simulink model "ASM_Traffic_V2X_Complete_Model_2"  (R2019a)
settings: Solver=ode1  StartTime=SIM.tstart.v  StopTime=Inf  FixedStep=SIM.StepSize.v  RelTol=1e-3
PostLoadFcn:
  | if any(exist('dsrtsu_mdlpostloadfcn', 'file') ~= 0), dsrtsu_mdlpostloadfcn('Execute', bdroot); end
  | try, asm_mdl_postloadfcn(bdroot, 'UpdateModel', 2200); catch, disp(lasterr); end,
undefined symbols (not defined in the file): _SensorPnts_1, _SensorPnts_13, _SensorPnts_17, _SensorPnts_21, _SensorPnts_25, _SensorPnts_29, _SensorPnts_33, _SensorPnts_37, _SensorPnts_41, _SensorPnts_45, _SensorPnts_49, _SensorPnts_5, _SensorPnts_53, _SensorPnts_57, _SensorPnts_9, _to_, CPT, G5A, ITS, MDL, rad, s_to_rpm, SIM
libraries: simulink x169, ASM_VehicleDynamics_lib x126, ASM_Traffic_lib x83, ASM_Utils_lib x49, mdbs x45, ASM_Environment_lib x17, dspindex x12, dsaV2xLibraryAux x10, dsmpblib x6, dsaV2xAsn1Library x4, dsaV2xLibrary x4, ASM_BrakeHydraulics_lib x4
(part 12 of 36)

== system ASM_Traffic_V2X_Complete_Model_2/MDL/Environment/Maneuver/LastValues ==
  VehicleDynamics_Signals : Inport
  Driver_Signals : Inport  Port=2
  Road_Signals : Inport  Port=3
  Maneuver_RefSignals : Inport  Port=4
  AvoidAlgLoop_AccPed : Memory
  AvoidAlgLoop_BrakePed : Memory
  AvoidAlgLoop_ClutchPed : Memory
  AvoidAlgLoop_Gear : Memory
  AvoidAlgLoop_Steer{,1..4} (5 alike) : Memory
  Bus Creator3 : BusCreator  Inputs=9
  Bus Selector1 : BusSelector  OutputSignals=Steering.Angle_SteeringWheel[deg],Steering.Trq_SteeringWheel[Nm]
  Bus Selector2 : BusSelector  OutputSignals=Pos_AccPedal[%],Pos_BrakePedal[%],Pos_ClutchPedal[%],Gear[],Angle_SteeringWheel[deg],AutomaticTrmCtrlSignals.SelectorLever[-3T|-2P|-1R|0N|1D]
  Bus Selector3 : BusSelector  OutputSignals=Sw_SteeringMode_Maneuver[1Angle|2Trq]
  Bus Selector5 : BusSelector  OutputSignals=Road_ASMVeh.d_Total_Veh_Road[m],Road_ASMVeh.LaneIdx_Total_Veh_Road[]
  Multiport Switch : MultiPortSwitch  Inputs=2
  LastValues : Outport
  wires:
  Bus Selector5/1 -> AvoidAlgLoop_Steer1/1  "<d_Total_Veh_Road[m]>"
  Bus Selector5/2 -> AvoidAlgLoop_Steer2/1  "<LaneIdx_Total_Veh_Road[]>"
  Road_Signals/1 -> Bus Selector5/1
  Driver_Signals/1 -> Bus Selector2/1
  Bus Creator3/1 -> LastValues/1
  AvoidAlgLoop_Steer2/1 -> Bus Creator3/7  "LaneIdx_Total_Veh_Road_Last[]"
  AvoidAlgLoop_Steer1/1 -> Bus Creator3/6  "d_Total_Veh_Road_Last[m]"
  AvoidAlgLoop_Steer/1 -> Bus Creator3/5  "Angle_SteeringWheel_Last[deg]"
  AvoidAlgLoop_Gear/1 -> Bus Creator3/4  "Gear_Last[]"
  AvoidAlgLoop_ClutchPed/1 -> Bus Creator3/3  "Pos_ClutchPedal_Last[%]"
  AvoidAlgLoop_BrakePed/1 -> Bus Creator3/2  "Pos_BrakePedal_Last[%]"
  AvoidAlgLoop_AccPed/1 -> Bus Creator3/1  "Pos_AccPedal_Last[%]"
  Bus Selector2/1 -> AvoidAlgLoop_AccPed/1  "<Pos_AccPedal[%]>"
  Bus Selector2/2 -> AvoidAlgLoop_BrakePed/1  "<Pos_BrakePedal[%]>"
  Bus Selector2/3 -> AvoidAlgLoop_ClutchPed/1  "<Pos_ClutchPedal[%]>"
  Bus Selector2/4 -> AvoidAlgLoop_Gear/1  "<Gear[]>"
  VehicleDynamics_Signals/1 -> Bus Selector1/1
  AvoidAlgLoop_Steer3/1 -> Bus Creator3/8  "Trq_SteeringWheel_Last[Nm]"
  Bus Selector1/2 -> AvoidAlgLoop_Steer3/1  "<Trq_SteeringWheel[Nm]>"
  Bus Selector2/5 -> Multiport Switch/2  "<Angle_SteeringWheel[deg]>"
  Maneuver_RefSignals/1 -> Bus Selector3/1
  Bus Selector3/1 -> Multiport Switch/1  "<Sw_SteeringMode_Maneuver[1Angle|2Trq]>"
  Multiport Switch/1 -> AvoidAlgLoop_Steer/1
  Bus Selector1/1 -> Multiport Switch/3  "<Angle_SteeringWheel[deg]>"
  AvoidAlgLoop_Steer4/1 -> Bus Creator3/9  "SelectorLever_Last[]"
  Bus Selector2/6 -> AvoidAlgLoop_Steer4/1  "<SelectorLever[-3T|-2P|-1R|0N|1D]>"

== system ASM_Traffic_V2X_Complete_Model_2/MDL/Environment/Maneuver/ParkingBrake ==
  Sw_ParkingBrake[0Off|1On] : Inport
  Bus Creator : BusCreator  Inputs=1
  ParkingBrakeSignals : Outport
  wires:
  Sw_ParkingBrake[0Off|1On]/1 -> Bus Creator/1  "Sw_ParkingBrake[0Off|1On]"
  Bus Creator/1 -> ParkingBrakeSignals/1  "ParkingBrakeSignals"

== system ASM_Traffic_V2X_Complete_Model_2/MDL/Environment/Maneuver/ReplaceBrake ==
  RefSignals_In : Inport
  Info : Inport  Port=2
  Bus Creator : BusCreator  Inputs=15
  Bus Selector : BusSelector  OutputSignals=Pos_AccPedal_Maneuver[%],Pos_BrakePedal_Maneuver[%],Pos_ClutchPedal_Maneuver[%],Gear_Maneuver[],Angle_SteeringWheel_Maneuver[deg],v_Vehicle_Ref_Maneuver[m|s],d_Maneuver[m],LaneIdx_Maneuver[],Dist_Def_Maneuver[],v_Vehicle_Ref_Preview_Maneuver[m|s],v_Vehicle_Ref_Preview_State[0Invalid|1CurrentSeg|2NextSeg],Sw_SteeringMode_Maneuver[1Angle|2Trq],Trq_Steering_Maneuver[Nm],SelectorLever_Maneuver[],Dist_Def_Refline_Maneuver[]
  Bus Selector4 : BusSelector  OutputSignals=ManeuverState[]
  Const_Replace_Pos_BrakePedal[%] : Constant  Value=65
  Multiport Switch : MultiPortSwitch  DataPortOrder=Zero-based contiguous  Inputs=2  zeroidx=on
  ReplaceEnable : Subsystem
  RefSignals : Outport
  wires:
  Bus Selector/15 -> Bus Creator/15  "<Dist_Def_Refline_Maneuver[]>"
  Bus Selector/14 -> Bus Creator/14  "<SelectorLever_Maneuver[]>"
  Bus Selector/13 -> Bus Creator/13  "<Trq_Steering_Maneuver[Nm]>"
  Bus Selector/12 -> Bus Creator/12  "<Sw_SteeringMode_Maneuver[1Angle|2Trq]>"
  Bus Selector/11 -> Bus Creator/11  "<v_Vehicle_Ref_Preview_State[0Invalid|1CurrentSeg|2NextSeg]>"
  Bus Selector/10 -> Bus Creator/10  "<v_Vehicle_Ref_Preview_Maneuver[m|s]>"
  Bus Selector/9 -> Bus Creator/9  "<Dist_Def_Maneuver[]>"
  Bus Selector/8 -> Bus Creator/8  "<LaneIdx_Maneuver[]>"
  Bus Selector/7 -> Bus Creator/7  "<d_Maneuver[m]>"
  [TAG_Sw_MasterBrakeCylinder_Mode] -> ReplaceEnable/2(Sw_MasterBrakeCylinder_Mode[1linear|2physical])
  Bus Selector4/1 -> ReplaceEnable/1(ManeuverState)  "<ManeuverState[]>"
  Info/1 -> Bus Selector4/1
  Multiport Switch/1 -> Bus Creator/2  "Pos_BrakePedal_Maneuver[%]"
  Const_Replace_Pos_BrakePedal[%]/1 -> Multiport Switch/3
  Bus Selector/2 -> Multiport Switch/2  "<Pos_BrakePedal_Maneuver[%]>"
  Bus Creator/1 -> RefSignals/1  "RefSignals"
  Bus Selector/6 -> Bus Creator/6  "<v_Vehicle_Ref_Maneuver[m|s]>"
  Bus Selector/5 -> Bus Creator/5  "<Angle_SteeringWheel_Maneuver[deg]>"
  Bus Selector/4 -> Bus Creator/4  "<Gear_Maneuver[]>"
  Bus Selector/3 -> Bus Creator/3  "<Pos_ClutchPedal_Maneuver[%]>"
  Bus Selector/1 -> Bus Creator/1  "<Pos_AccPedal_Maneuver[%]>"
  RefSignals_In/1 -> Bus Selector/1
  ReplaceEnable/1(ReplaceEnable[0Off|1On]) -> Multiport Switch/1

== system ASM_Traffic_V2X_Complete_Model_2/MDL/Environment/Maneuver/ReplaceSelectorLever_Mode ==
  ModeSignals_In : Inport
  Bus Creator : BusCreator  Inputs=10
  Bus Selector : BusSelector  OutputSignals=AccBr_Mode[1Stim|2Driver],GearClutch_Mode[1Stim|2Driver|3OpenClutch|4RefGear],Steer_Mode[1Stim|2Driver|3Fix],Road_Mode[1NoRoad|2Straight|3Circle|4Road],LatDriver[1LatCtrl1|2LatCtrl2],LatCtrl_Mode[1Pos|2Yaw],AdaptVelocityToRoad_Mode[1Off|2On],ForceToRoad_Mode[1Off|2On],CurvatureCalculation_Mode[1Road|2Driver],SelectorLever_Mode[1Stim|2Driver]
  Multiport Switch : MultiPortSwitch  Inputs=2  DiagnosticForDefault=Warning
  Selector1 : Selector  InputPortWidth=4  IndexOptions=Index vector (dialog)  Indices=[3]  OutputSizes=1
  ModeSignals : Outport
  wires:
  Bus Creator/1 -> ModeSignals/1  "ModeSignals"
  ModeSignals_In/1 -> Bus Selector/1
  [TAG_Sw_ManeuverControl] -> Selector1/1
  Bus Selector/1 -> Bus Creator/1  "<AccBr_Mode[1Stim|2Driver]>"
  Bus Selector/2 -> Bus Creator/2  "<GearClutch_Mode[1Stim|2Driver|3OpenClutch|4RefGear]>"
  Bus Selector/3 -> Bus Creator/3  "<Steer_Mode[1Stim|2Driver|3Fix]>"
  Bus Selector/4 -> Bus Creator/4  "<Road_Mode[1NoRoad|2Straight|3Circle|4Road]>"
  Bus Selector/5 -> Bus Creator/5  "<LatDriver[1LatCtrl1|2LatCtrl2]>"
  Bus Selector/6 -> Bus Creator/6  "<LatCtrl_Mode[1Pos|2Yaw]>"
  Bus Selector/7 -> Bus Creator/7  "<AdaptVelocityToRoad_Mode[1Off|2On]>"
  Bus Selector/8 -> Bus Creator/8  "<ForceToRoad_Mode[1Off|2On]>"
  Selector1/1 -> Multiport Switch/1  "Sw_ManualDriving[1ManSched|2Manual]"
  [TAG_SW_SelectorLever_Mode] -> Multiport Switch/3  "SelectorLever_Mode[1Stim|2Driver]"
  Bus Selector/10 -> Multiport Switch/2  "<SelectorLever_Mode[1Stim|2Driver]>"
  Multiport Switch/1 -> Bus Creator/10  "SelectorLever_Mode[1Stim|2Driver]"
  Bus Selector/9 -> Bus Creator/9  "<CurvatureCalculation_Mode[1Road|2Driver]>"

== system ASM_Traffic_V2X_Complete_Model_2/MDL/Environment/Maneuver/Reset _IfModeSwitched ==
  DrvTrnMode : Inport
  TrmMode : Inport  Port=2
  TireMode : Inport  Port=3
  DTC{1..4} (4 alike) : DataTypeConversion  SaturateOnIntegerOverflow=on  RndMeth=Zero
  Gain_DrvTrnMode : Gain  SaturateOnIntegerOverflow=on  OutDataTypeStr=Inherit: Same as input  ParamDataTypeStr=Inherit: Same as input
  Gain_TireMode : Gain  SaturateOnIntegerOverflow=on  OutDataTypeStr=Inherit: Same as input  ParamDataTypeStr=Inherit: Same as input
  Gain_Total : Gain  SaturateOnIntegerOverflow=on  OutDataTypeStr=Inherit: Same as input  ParamDataTypeStr=Inherit: Same as input
  Gain_TrmMode : Gain  SaturateOnIntegerOverflow=on  OutDataTypeStr=Inherit: Same as input  ParamDataTypeStr=Inherit: Same as input
  IgnoreSimulationStart : Subsystem
  LogOp_Reset : Logic  Operator=OR  Inputs=3  AllPortsSameDT=off
  Mem_DrvTrnMode : Memory
  Mem_TireMode : Memory
  Mem_TrmMode : Memory
  RelOp_DrvTrnMode : RelationalOperator  Operator=~=  RndMeth=Nearest
  RelOp_TireMode : RelationalOperator  Operator=~=  RndMeth=Nearest
  RelOp_TrmMode : RelationalOperator  Operator=~=  RndMeth=Nearest
  Sat_DrvTrnMode : Saturate  UpperLimit=3  LowerLimit=1
  Sat_TireMode : Saturate  UpperLimit=2  LowerLimit=1
  Sat_TrmMode : Saturate  UpperLimit=2  LowerLimit=1
  Reset_IfModeSwitched : Outport
  wires:
  DrvTrnMode/1 -> Sat_DrvTrnMode/1
  Sat_DrvTrnMode/1 -> Mem_DrvTrnMode/1, RelOp_DrvTrnMode/2
  Mem_DrvTrnMode/1 -> RelOp_DrvTrnMode/1
  IgnoreSimulationStart/1(Reset_Out) -> Gain_Total/1
  Gain_Total/1 -> Reset_IfModeSwitched/1
  Sat_TrmMode/1 -> RelOp_TrmMode/2, Mem_TrmMode/1
  Mem_TrmMode/1 -> RelOp_TrmMode/1
  Sat_TireMode/1 -> Mem_TireMode/1, RelOp_TireMode/2
  Mem_TireMode/1 -> RelOp_TireMode/1
  TrmMode/1 -> Sat_TrmMode/1
  TireMode/1 -> Sat_TireMode/1
  RelOp_DrvTrnMode/1 -> DTC1/1
  RelOp_TrmMode/1 -> DTC2/1
  RelOp_TireMode/1 -> DTC3/1
  Gain_DrvTrnMode/1 -> LogOp_Reset/1
  Gain_TrmMode/1 -> LogOp_Reset/2
  Gain_TireMode/1 -> LogOp_Reset/3
  LogOp_Reset/1 -> DTC4/1
  DTC1/1 -> Gain_DrvTrnMode/1
  DTC2/1 -> Gain_TrmMode/1
  DTC3/1 -> Gain_TireMode/1
  DTC4/1 -> IgnoreSimulationStart/1(Reset_In)

== system ASM_Traffic_V2X_Complete_Model_2/MDL/Environment/Maneuver/SimulationControl ==
  VehicleDynamics_Signals : Inport
  Bus Selector4 : BusSelector  OutputSignals=VehicleMovement.Positions.Angle_Vehicle_CoorSys_E[x;y;z][deg].Angle_Roll_Vehicle_CoorSys_E[deg],VehicleMovement.Positions.Angle_Vehicle_CoorSys_E[x;y;z][deg].Angle_Pitch_Vehicle_CoorSys_E[deg]
  KeepVehiclePosition : Subsystem
  Keep_VehiclePosition[0|1] : Outport
  wires:
  KeepVehiclePosition/1(Keep_VehiclePosition[0|1]) -> Keep_VehiclePosition[0|1]/1
  Bus Selector4/1 -> KeepVehiclePosition/1(Angle_Roll_Vehicle_CoorSys_E[deg])  "<Angle_Roll_Vehicle_CoorSys_E[deg]>"
  Bus Selector4/2 -> KeepVehiclePosition/2(Angle_Pitch_Vehicle_CoorSys_E[deg])  "<Angle_Pitch_Vehicle_CoorSys_E[deg]>"
  VehicleDynamics_Signals/1 -> Bus Selector4/1

== system ASM_Traffic_V2X_Complete_Model_2/MDL/Environment/Maneuver/StartButton ==
  StartButton_ManSched[0Off|1On] : Inport
  StartButton_Signals_ : Inport  Port=2
  Bus Creator : BusCreator  Inputs=1
  Bus Selector : BusSelector  OutputSignals=Sw_StartButton[0Off|1On],Sw_StartButton_Mode[1Manual|2ManSched]
  Manual : simulink/Logic and Bit Operations/Compare To Constant  relop===  const=1  OutDataTypeStr=boolean
  Switch : Switch  Criteria=u2 ~= 0
  StartButton_Signals : Outport
  wires:
  StartButton_ManSched[0Off|1On]/1 -> Switch/3
  Manual/1 -> Switch/2
  Bus Creator/1 -> StartButton_Signals/1  "StartButtonSignals"
  Switch/1 -> Bus Creator/1  "Sw_StartButton[0Off|1On]"
  Bus Selector/2 -> Manual/1  "<Sw_StartButton_Mode[1Manual|2ManSched]>"
  Bus Selector/1 -> Switch/1  "<Sw_StartButton[0Off|1On]>"
  StartButton_Signals_/1 -> Bus Selector/1

== system ASM_Traffic_V2X_Complete_Model_2/MDL/Environment/Maneuver/Testbench ==
  SW_Testbench[0Off|1On] : Inport
  n_Engine_Set[rpm] : Inport  Port=2
  Bus Creator : BusCreator  Inputs=2
  Testbench : Outport
  wires:
  SW_Testbench[0Off|1On]/1 -> Bus Creator/1  "SW_Testbench[0Off|1On]"
  Bus Creator/1 -> Testbench/1  "Testbench"
  n_Engine_Set[rpm]/1 -> Bus Creator/2  "n_Engine_Set[rpm]"

== system ASM_Traffic_V2X_Complete_Model_2/MDL/Environment/Maneuver/TipShift ==
  SW_TipTronic[-1Down|0Off|1Up] : Inport
  Bus Creator : BusCreator  Inputs=1
  TipShiftSignals : Outport
  wires:
  SW_TipTronic[-1Down|0Off|1Up]/1 -> Bus Creator/1  "SW_TipTronic[-1Down|0Off|1Up]"
  Bus Creator/1 -> TipShiftSignals/1  "TipShiftSignals"

== system ASM_Traffic_V2X_Complete_Model_2/MDL/Environment/Maneuver/VehicleInitStates ==
  note: Set v_x_Init to zero if Keep_VehiclePosition is enabled or the maneuver state is BRAKE or WAIT.
  note: Use v_x_Init from VehicleInitStates_External if the maneuver state is INIT_MANUAL or MANUAL; else use v_x_Init from the maneuver scheduler.
  Keep_VehiclePosition[0|1] : Inport
  ManeuverState[] : Inport  Port=2
  v_Vehicle_Init_Mnv[km|h] : Inport  Port=3
  VehicleInitStates_External : Inport  Port=4
  Bus Creator1 : BusCreator  Inputs=1
  Const_zero_v_x_Init[km|h] : Constant  Value=0  VectorParams1D=off
  Data Type Conversion1 : DataTypeConversion  OutDataTypeStr=double
  Demux : Demux  Outputs=[1 1 1 3]
  Keep_VehiclePosition_enabled : simulink/Logic and Bit Operations/Compare To Constant  relop===  const=1  OutDataTypeStr=uint8  ZeroCross=off
  Logical Operator3 : Logic  Operator=OR  Inputs=3  AllPortsSameDT=off  OutDataTypeStr=boolean
  Logical Operator4 : Logic  Operator=OR  AllPortsSameDT=off  OutDataTypeStr=boolean
  Multiport Switch1 : MultiPortSwitch  DataPortOrder=Zero-based contiguous  Inputs=2  zeroidx=on
  Multiport Switch2 : MultiPortSwitch  DataPortOrder=Zero-based contiguous  Inputs=2  zeroidx=on
  Mux : Mux  Inputs=3
  Mux1 : Mux  Inputs=[3 3]
  State_BRAKE : simulink/Logic and Bit Operations/Compare To Constant  relop===  const=4  OutDataTypeStr=uint8  ZeroCross=off
  State_INIT_MANUAL : simulink/Logic and Bit Operations/Compare To Constant  relop===  const=6  OutDataTypeStr=uint8  ZeroCross=off
  State_MANUAL : simulink/Logic and Bit Operations/Compare To Constant  relop===  const=7  OutDataTypeStr=uint8  ZeroCross=off
  State_WAIT : simulink/Logic and Bit Operations/Compare To Constant  relop===  const=5  OutDataTypeStr=uint8  ZeroCross=off
  Sw_KeepVehiclePosition_Dependency : Gain
  Sw_ManeuverState_Dependency : Gain
  Unit Delay : UnitDelay  SampleTime=-1
  UnitConversion : ASM_Utils_lib/UnitConversion/UnitConversion  Selection=km/h_to_m/s
  VehicleInitStates : Outport
  wires:
  Demux/3 -> Mux/3  "vz"
  Demux/2 -> Mux/2  "vy"
  Bus Creator1/1 -> VehicleInitStates/1  "VehicleInitStates"
  Mux/1 -> UnitConversion/1
  Demux/4 -> Mux1/2  "w_Init[x;y;z][rad|s]"
  ManeuverState[]/1 -> Sw_ManeuverState_Dependency/1
  Unit Delay/1 -> Mux/1  "vx"
  Mux1/1 -> Bus Creator1/1  "q_dt_Vehicle_Init[6x1]"
  Demux/1 -> Multiport Switch2/3
  State_BRAKE/1 -> Logical Operator3/2
  State_WAIT/1 -> Logical Operator3/3
  Sw_ManeuverState_Dependency/1 -> State_BRAKE/1, State_WAIT/1, State_INIT_MANUAL/1, State_MANUAL/1
  Keep_VehiclePosition[0|1]/1 -> Sw_KeepVehiclePosition_Dependency/1
  Sw_KeepVehiclePosition_Dependency/1 -> Keep_VehiclePosition_enabled/1
  Keep_VehiclePosition_enabled/1 -> Logical Operator3/1
  Logical Operator3/1 -> Data Type Conversion1/1
  Data Type Conversion1/1 -> Multiport Switch1/1
  Const_zero_v_x_Init[km|h]/1 -> Multiport Switch1/3
  Multiport Switch2/1 -> Multiport Switch1/2
  Multiport Switch1/1 -> Unit Delay/1
  State_INIT_MANUAL/1 -> Logical Operator4/1
  State_MANUAL/1 -> Logical Operator4/2
  Logical Operator4/1 -> Multiport Switch2/1
  v_Vehicle_Init_Mnv[km|h]/1 -> Multiport Switch2/2
  VehicleInitStates_External/1 -> Demux/1
  UnitConversion/1 -> Mux1/1  "v_Init[x;y;z][m|s]"

== system ASM_Traffic_V2X_Complete_Model_2/MDL/Environment/Road/ASMSignalCollector ==
  SwitchRoad[0BasicRoad|1StandardRoad] : Inport
  Bus Creator : BusCreator  Inputs=11
  Bus Creator1 : BusCreator  Inputs=2
  Bus Selector1 : BusSelector  OutputSignals=Road_Init,Road_ASMVeh,Road_ContactPoints,Road_Preview  OutputAsBus=on
  Bus Selector2 : BusSelector  OutputSignals=Road_Info,Road_TrafficFellows,UserSignals
  Bus Selector4 : BusSelector  OutputSignals=Road_Init,Road_ASMVeh,Road_ContactPoints,Road_Preview
  Switch1 : Switch  Threshold=0.5
  tag scope: ASMBUS_Environment_Road=global
  wires:
  Bus Creator1/1 -> Bus Creator/11  "LaneSensor_Dynamic"
  [ASMBUS_Environment_LaneSensor_Dynamic_Output] -> Bus Creator1/2  "Sensor_Output"
  [ASMBUS_Environment_LaneSensor_Dynamic_Parameters] -> Bus Creator1/1  "Parameters"
  [ASMBUS_Environment_Ambient] -> Bus Creator/10
  [ASMBUS_Environment_Customized_UserSignals] -> Bus Creator/8
  [ASMBUS_Environment_PosVehGPS] -> Bus Creator/9
  Bus Selector2/2 -> Bus Creator/6  "<Road_TrafficFellows>"
  Bus Selector2/3 -> Bus Creator/7  "<UserSignals>"
  Bus Selector2/1 -> Bus Creator/5  "<Road_Info>"
  Bus Selector4/4 -> Bus Creator/4  "<Road_Preview>"
  Bus Selector4/3 -> Bus Creator/3  "<Road_ContactPoints>"
  Bus Selector4/2 -> Bus Creator/2  "<Road_ASMVeh>"
  Bus Selector4/1 -> Bus Creator/1  "<Road_Init>"
  [ASMBUS_Environment_StandardRoad] -> Bus Selector1/1, Bus Selector2/1
  [ASMBUS_Environment_BasicRoads] -> Switch1/3
  Bus Selector1/1 -> Switch1/1
  SwitchRoad[0BasicRoad|1StandardRoad]/1 -> Switch1/2
  Switch1/1 -> Bus Selector4/1
  Bus Creator/1 -> [ASMBUS_Environment_Road]  "Road"

== system ASM_Traffic_V2X_Complete_Model_2/MDL/Environment/Road/Customize_UserSignals ==
  UserSignals_In : Inport
  Bus Creator : BusCreator  Inputs=3
  Bus Selector1 : BusSelector  OutputSignals=User1[],User2[],User3[]
  CustomizedUserSignals : Subsystem
  ASMSignalBus : Outport
  UserSignals_Customized : Outport  Port=2
  wires:
  UserSignals_In/1 -> Bus Selector1/1
  Bus Creator/1 -> UserSignals_Customized/1, ASMSignalBus/1  "UserSignals_Customized"
  Bus Selector1/1 -> CustomizedUserSignals/1(User1[])  "<User1[]>"
  Bus Selector1/2 -> CustomizedUserSignals/2(User2[])  "<User2[]>"
  Bus Selector1/3 -> CustomizedUserSignals/3(User3[])  "<User3[]>"
  CustomizedUserSignals/1(GPS_Method[]) -> Bus Creator/1
  CustomizedUserSignals/2(Const_Offset_Lat[deg]) -> Bus Creator/2
  CustomizedUserSignals/3(Const_Offset_Long[deg]) -> Bus Creator/3

== system ASM_Traffic_V2X_Complete_Model_2/MDL/Environment/Road/SignalRouting ==
  SwitchRoad[0BasicRoad|1StandardRoad] : Inport
  BasicRoad : Inport  Port=2
  StandardRoad : Inport  Port=3
  Info : Inport  Port=4
  TrafficFellows : Inport  Port=5
  UserSignals : Inport  Port=6
  TrafficObject_Data : Inport  Port=7
  Customized_UserSignals : Inport  Port=8
  Pos_Vehicle_GPS[Long;Lat][deg] : Inport  Port=9
  Ambient : Inport  Port=10
  LaneSensor_Dynamic : Inport  Port=11
  Bus Creator3 : BusCreator  Inputs=12
  Bus Selector1 : BusSelector  OutputSignals=Road_Init,Road_ASMVeh,Road_ContactPoints,Road_Preview
  Mapping_CP : Subsystem
  Switch1 : Switch  Threshold=0.5
  Unit Delay : UnitDelay  SampleTime=-1
  Road : Outport
  wires:
  LaneSensor_Dynamic/1 -> Bus Creator3/12
  TrafficObject_Data/1 -> Bus Creator3/8
  TrafficFellows/1 -> Bus Creator3/6
  UserSignals/1 -> Bus Creator3/7
  Pos_Vehicle_GPS[Long;Lat][deg]/1 -> Bus Creator3/10
  Ambient/1 -> Bus Creator3/11
  Customized_UserSignals/1 -> Bus Creator3/9
  BasicRoad/1 -> Switch1/3
  StandardRoad/1 -> Switch1/1
  SwitchRoad[0BasicRoad|1StandardRoad]/1 -> Switch1/2
  Switch1/1 -> Bus Selector1/1
  Bus Creator3/1 -> Road/1  "Road"
  Bus Selector1/2 -> Bus Creator3/2  "<Road_ASMVeh>"
  Bus Selector1/3 -> Mapping_CP/1(In1)  "<Road_ContactPoints>"
  Bus Selector1/4 -> Bus Creator3/4  "<Road_Preview>"
  Info/1 -> Bus Creator3/5
  Mapping_CP/1(Out1) -> Bus Creator3/3  "Road_ContactPoints"
  Bus Selector1/1 -> Unit Delay/1  "<Road_Init>"
  Unit Delay/1 -> Bus Creator3/1  "Road_InitialStates"

== system ASM_Traffic_V2X_Complete_Model_2/MDL/Environment/Road/distance2TargetLaneLines ==
  posVeh_y : Inport
  Input : Inport  Port=2
  Abs{,1..3} (4 alike) : Abs
  Bus Selector : BusSelector  OutputSignals=CurrentLane.LeftSide.Distance_Marker_Left[m],CurrentLane.RightSide.Distance_Marker_Right[m],CurrentLane.Common.LaneID_PrefLane[]
  LeftLine_position : Constant  Value=-5.25
  RightLine_position : Constant  Value=-8.75
  Subtract : Sum  Inputs=+-
  Subtract1 : Sum  Inputs=+-
  LeftLineDistance : Outport
  RightLineDistance : Outport  Port=2
  Right : Outport  Port=3
  Left : Outport  Port=4
  Lane_ID : Outport  Port=5
  wires:
  Input/1 -> Abs1/1, Abs/1
  LeftLine_position/1 -> Abs2/1
  Abs2/1 -> Subtract1/1
  Abs1/1 -> Subtract1/2
  RightLine_position/1 -> Abs3/1
  Abs3/1 -> Subtract/1
  Abs/1 -> Subtract/2
  Subtract/1 -> Right/1
  Subtract1/1 -> Left/1
  posVeh_y/1 -> Bus Selector/1
  Bus Selector/1 -> LeftLineDistance/1  "<Distance_Marker_Left[m]>"
  Bus Selector/2 -> RightLineDistance/1  "<Distance_Marker_Right[m]>"
  Bus Selector/3 -> Lane_ID/1  "<LaneID_PrefLane[]>"

== system ASM_Traffic_V2X_Complete_Model_2/MDL/Environment/Traffic/ASMSignalCollector ==
  Bus Creator1 : BusCreator  Inputs=3
  tag scope: ASMBUS_Environment_Traffic=global
  wires:
  Bus Creator1/1 -> [ASMBUS_Environment_Traffic]  "Traffic"
  [ASMBUS_Environment_Traffic_FellowMovement] -> Bus Creator1/1
  [ASMBUS_Environment_Traffic_ObjectParameters] -> Bus Creator1/2
  [ASMBUS_Environment_Traffic_Sensors] -> Bus Creator1/3

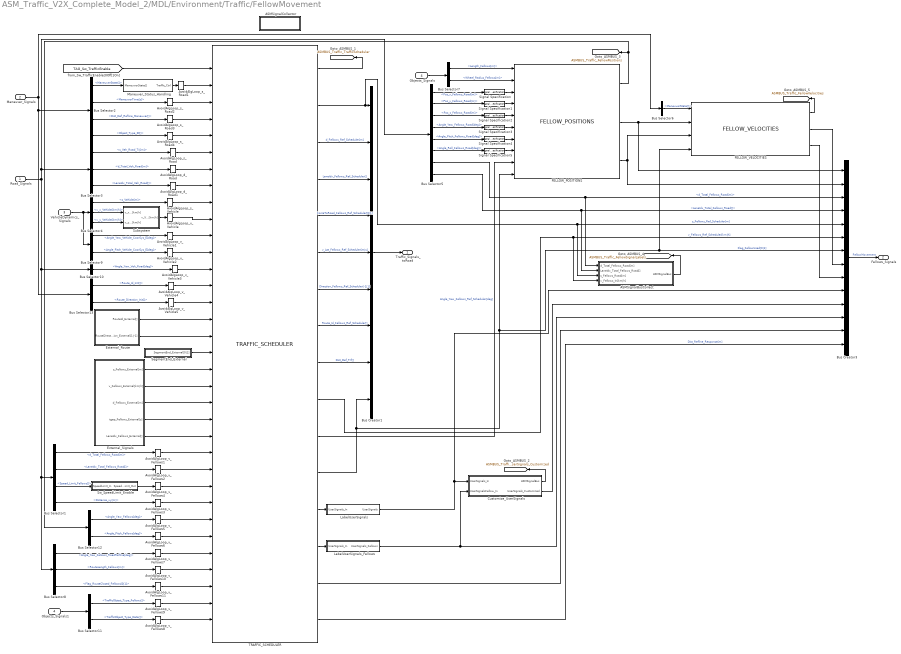
== system ASM_Traffic_V2X_Complete_Model_2/MDL/Environment/Traffic/FellowMovement ==
  Road_Signals : Inport
  Maneuver_Signals : Inport  Port=2
  VehicleDynamics_Signals : Inport  Port=3
  Objects_Signals : Inport  Port=4
  ASMSignalBusCollect : Subsystem
  ASMSignalCollector : Subsystem
  AvoidAlgLoop_d_Road : Memory
  AvoidAlgLoop_d_Road1 : Memory
  AvoidAlgLoop_s_Road{,1..4} (5 alike) : Memory
  AvoidAlgLoop_s_Vehicle : Memory
  AvoidAlgLoop_v_Fellows{1..11} (11 alike) : Memory
  AvoidAlgLoop_v_Vehicle{,1..5} (6 alike) : Memory
  Bus Creator1 : BusCreator  Inputs=9
  Bus Creator3 : BusCreator  Inputs=14
  Bus Selector1 : BusSelector  OutputSignals=Road_TrafficFellows.d_Total_Fellows_Road[m],Road_TrafficFellows.LaneIdx_Total_Fellows_Road[],Road_TrafficFellows.Speed_Limit_Fellows[],Road_TrafficFellows.Dist_Response_Traffic.Distance_xy[m]
  Bus Selector10 : BusSelector  OutputSignals=Road_ASMVeh.Angle_Yaw_Veh_Road[deg]
  Bus Selector11 : BusSelector  OutputSignals=TrafficObject_Type_Fellows[],TrafficObject_Type_Data[]
  Bus Selector12 : BusSelector  OutputSignals=Angle_Fellows[x;y;z][deg].Angle_Yaw_Fellows[deg],Angle_Fellows[x;y;z][deg].Angle_Pitch_Fellows[deg]
  Bus Selector13 : BusSelector  OutputSignals=InitialVehStates.Route_Id_Init[],InitialVehStates.Route_Direction_Init[]
  Bus Selector2 : BusSelector  OutputSignals=Info.ManeuverState[],Info.ManeuverTime[s],RefSignals.Dist_Def_Refline_Maneuver[],Parameters.Object_Type_ID[]
  Bus Selector3 : BusSelector  OutputSignals=Road_ASMVeh.s_Veh_Road_Trj[m],Road_ASMVeh.d_Total_Veh_Road[m],Road_ASMVeh.LaneIdx_Total_Veh_Road[]
  Bus Selector4 : BusSelector  OutputSignals=VehicleMovement.Positions.s_Vehicle[m],VehicleMovement.Velocities.v_x_Vehicle[km|h],VehicleMovement.Velocities.v_y_Vehicle[km|h]
  Bus Selector5 : BusSelector  OutputSignals=Road_TrafficFellows.Pos_x_Fellows_Road[m],Road_TrafficFellows.Pos_y_Fellows_Road[m],Road_TrafficFellows.Pos_z_Fellows_Road[m],Road_TrafficFellows.Angle_Yaw_Fellows_Road[deg],Road_TrafficFellows.Angle_Pitch_Fellows_Road[deg],Road_TrafficFellows.Angle_Roll_Fellows_Road[deg],Road_TrafficFellows.d_Total_Fellows_Road[m],Road_TrafficFellows.LaneIdx_Total_Fellows_Road[]
  Bus Selector6 : BusSelector  OutputSignals=Info.ManeuverState[]
  Bus Selector7 : BusSelector  OutputSignals=FellowsGeometry.Size_Fellows[m].Length_Fellows[m],FellowsGeometry.Wheel_Radius_Fellows[m]
  Bus Selector8 : BusSelector  OutputSignals=Road_TrafficFellows.Angle_Yaw_Fellows_RoadRefline[deg],Road_TrafficFellows.RouteLength_Fellows[m],Road_TrafficFellows.Flag_RouteClosed_Fellows[0|1]
  Bus Selector9 : BusSelector  OutputSignals=VehicleMovement.Positions.Angle_Vehicle_CoorSys_E[x;y;z][deg].Angle_Yaw_Vehicle_CoorSys_E[deg],VehicleMovement.Positions.Angle_Vehicle_CoorSys_E[x;y;z][deg].Angle_Pitch_Vehicle_CoorSys_E[deg]
  Customize_UserSignals : Subsystem
  External_Route : Subsystem
  External_Signals : Subsystem
  FELLOW_POSITIONS : ASM_Traffic_lib/Movement/FELLOW_POSITIONS  StepSize=SIM.StepSize  ASMProperties=struct('Name','FELLOW_POSITIONS','Version','6.0','Library','ASM_Traffic_lib')
  FELLOW_VELOCITIES : ASM_Traffic_lib/Movement/FELLOW_VELOCITIES  ASMProperties=struct('Name','FELLOW_VELOCITIES','Version','1.0','Library','ASM_Traffic_lib')  ASMInstanceName=fellow_velocities  ASMInstanceID=1
  LabelUserSignals : Subsystem
  LabelUserSignals_Fellows : Subsystem
  Maneuver_Status_Handling : Subsystem
  Objects_Signals1 : InportShadow  Port=4
  SegmentEnd_External : Subsystem
  Signal Specification{,1..5} (6 alike) : SignalSpecification  Dimensions=MDL.Traffic.MaxNumFellows.v
  Subsystem : Subsystem
  Sw_SpeedLimit_Enable : Subsystem
  TRAFFIC_SCHEDULER : ASM_Traffic_lib/Movement/TRAFFIC_SCHEDULER  Tag=ASM_SUBCOMPONENT  TrafficVector=MDL.Traffic.TrafficScheduler.Scenario  MaxNumFellows=MDL.Traffic.MaxNumFellows  MaxNumFDUserSignals=MDL.Traffic.MaxNumFDUserSignals  MaxNumUserSignals=MDL.Traffic.MaxNumUserSignals  ASMProperties=struct('Name','TRAFFIC_SCHEDULER','Version','18.0','Library','ASM_Traffic_lib')  ASMInstanceName=traffic_scheduler  ASMInstanceID=1
  Traffic_Signals_toRoad : Outport
  Fellows_Signals : Outport  Port=2
  tag scope: ASMBUS_Traffic_FellowPositions=global, ASMBUS_Traffic_FellowSignalLabels=global, ASMBUS_Traffic_FellowVelocities=global, ASMBUS_Traffic_TrafficScheduler=global, ASMBUS_Traffic_UserSignals_Customized=global
  wires:
  AvoidAlgLoop_v_Fellows9/1 -> TRAFFIC_SCHEDULER/33
  AvoidAlgLoop_v_Fellows11/1 -> TRAFFIC_SCHEDULER/32
  AvoidAlgLoop_v_Fellows10/1 -> TRAFFIC_SCHEDULER/31
  AvoidAlgLoop_v_Fellows7/1 -> TRAFFIC_SCHEDULER/30
  AvoidAlgLoop_v_Fellows6/1 -> TRAFFIC_SCHEDULER/29
  AvoidAlgLoop_v_Fellows5/1 -> TRAFFIC_SCHEDULER/28
  AvoidAlgLoop_v_Fellows3/1 -> TRAFFIC_SCHEDULER/27
  AvoidAlgLoop_v_Fellows4/1 -> TRAFFIC_SCHEDULER/26
  AvoidAlgLoop_v_Fellows2/1 -> TRAFFIC_SCHEDULER/25
  AvoidAlgLoop_v_Fellows1/1 -> TRAFFIC_SCHEDULER/24
  External_Signals/5(LaneIdx_Fellows_External[]) -> TRAFFIC_SCHEDULER/23
  External_Signals/4(tgap_Fellows_External[s]) -> TRAFFIC_SCHEDULER/22
  External_Signals/3(d_Fellows_External[m]) -> TRAFFIC_SCHEDULER/21
  External_Signals/2(v_Fellows_External[km|h]) -> TRAFFIC_SCHEDULER/20
  External_Signals/1(s_Fellows_External[m]) -> TRAFFIC_SCHEDULER/19
  SegmentEnd_External/1(SegmentEnd_External[0|1]) -> TRAFFIC_SCHEDULER/18
  External_Route/2(RouteDirection_External[1|-1]) -> TRAFFIC_SCHEDULER/17
  External_Route/1(RouteId_External[]) -> TRAFFIC_SCHEDULER/16
  Bus Selector13/2 -> AvoidAlgLoop_v_Vehicle5/1  "<Route_Direction_Init[]>"
  AvoidAlgLoop_v_Vehicle5/1 -> TRAFFIC_SCHEDULER/15
  AvoidAlgLoop_s_Road2/1 -> TRAFFIC_SCHEDULER/3
  AvoidAlgLoop_v_Fellows8/1 -> TRAFFIC_SCHEDULER/34
  AvoidAlgLoop_v_Vehicle4/1 -> TRAFFIC_SCHEDULER/14
  Bus Selector8/3 -> AvoidAlgLoop_v_Fellows11/1  "<Flag_RouteClosed_Fellows[0|1]>"
  Bus Selector8/2 -> AvoidAlgLoop_v_Fellows10/1  "<RouteLength_Fellows[m]>"
  AvoidAlgLoop_s_Road4/1 -> TRAFFIC_SCHEDULER/5
  AvoidAlgLoop_s_Road3/1 -> TRAFFIC_SCHEDULER/4
  AvoidAlgLoop_s_Road1/1 -> TRAFFIC_SCHEDULER/2
  AvoidAlgLoop_v_Vehicle3/1 -> TRAFFIC_SCHEDULER/13
  Bus Selector12/2 -> AvoidAlgLoop_v_Fellows6/1  "<Angle_Pitch_Fellows[deg]>"
  FELLOW_POSITIONS/1 -> Bus Selector12/1, [ASMBUS_Traffic_FellowPositions]
  Bus Selector13/1 -> AvoidAlgLoop_v_Vehicle4/1  "<Route_Id_Init[]>"
  Bus Selector10/1 -> AvoidAlgLoop_v_Vehicle3/1  "<Angle_Yaw_Veh_Road[deg]>"
  AvoidAlgLoop_v_Vehicle2/1 -> TRAFFIC_SCHEDULER/12
  AvoidAlgLoop_v_Vehicle1/1 -> TRAFFIC_SCHEDULER/11
  AvoidAlgLoop_v_Vehicle/1 -> TRAFFIC_SCHEDULER/10
  AvoidAlgLoop_s_Vehicle/1 -> TRAFFIC_SCHEDULER/9
  AvoidAlgLoop_d_Road1/1 -> TRAFFIC_SCHEDULER/8
  AvoidAlgLoop_d_Road/1 -> TRAFFIC_SCHEDULER/7
  AvoidAlgLoop_s_Road/1 -> TRAFFIC_SCHEDULER/6
  Bus Selector2/4 -> AvoidAlgLoop_s_Road4/1  "<Object_Type_ID[]>"
  Bus Selector2/3 -> AvoidAlgLoop_s_Road3/1  "<Dist_Def_Refline_Maneuver[]>"
  Bus Selector11/2 -> AvoidAlgLoop_v_Fellows8/1  "<TrafficObject_Type_Data[]>"
  Bus Selector11/1 -> AvoidAlgLoop_v_Fellows9/1  "<TrafficObject_Type_Fellows[]>"
  Objects_Signals1/1 -> Bus Selector11/1
  Bus Selector9/2 -> AvoidAlgLoop_v_Vehicle2/1  "<Angle_Pitch_Vehicle_CoorSys_E[deg]>"
  Bus Selector9/1 -> AvoidAlgLoop_v_Vehicle1/1  "<Angle_Yaw_Vehicle_CoorSys_E[deg]>"
  VehicleDynamics_Signals/1 -> Bus Selector4/1, Bus Selector9/1
  Bus Selector12/1 -> AvoidAlgLoop_v_Fellows5/1  "<Angle_Yaw_Fellows[deg]>"
  Bus Selector8/1 -> AvoidAlgLoop_v_Fellows7/1  "<Angle_Yaw_Fellows_RoadRefline[deg]>"
  TRAFFIC_SCHEDULER/16 -> Bus Creator3/14  "Dist_Refline_Response[m]"
  FELLOW_VELOCITIES/3 -> Bus Creator3/9
  FELLOW_VELOCITIES/2 -> Bus Creator3/8
  Bus Selector6/1 -> FELLOW_VELOCITIES/1  "<ManeuverState[]>"
  FELLOW_VELOCITIES/1 -> [ASMBUS_Traffic_FellowVelocities]
  Subsystem/1(v_Vehicle[km|h]) -> AvoidAlgLoop_v_Vehicle/1
  Bus Selector4/3 -> Subsystem/2(v_y_Vehicle[km|h])  "<v_y_Vehicle[km|h]>"
  Bus Selector4/2 -> Subsystem/1(v_x_Vehicle[km|h])  "<v_x_Vehicle[km|h]>"
  ASMSignalBusCollect/1(ASMSignalBus) -> [ASMBUS_Traffic_FellowSignalLabels]
  TRAFFIC_SCHEDULER/1 -> [ASMBUS_Traffic_TrafficScheduler]
  LabelUserSignals_Fellows/1(UserSignals_Fellows) -> Customize_UserSignals/2(UserSignalsFellow_In), Bus Creator3/12
  LabelUserSignals/1(UserSignals) -> Customize_UserSignals/1(UserSignals_In), Bus Creator3/10
  Customize_UserSignals/2(UserSignals_Customized) -> Bus Creator3/11
  FELLOW_POSITIONS/3 -> Bus Creator3/2, FELLOW_VELOCITIES/3
  FELLOW_POSITIONS/2 -> Bus Creator3/1, FELLOW_VELOCITIES/2
  Bus Selector5/8 -> Bus Creator3/4, ASMSignalBusCollect/2(LaneIdx_Total_Fellows_Road[])  "<LaneIdx_Total_Fellows_Road[]>"
  Bus Selector5/7 -> Bus Creator3/3, ASMSignalBusCollect/1(d_Total_Fellows_Road[m])  "<d_Total_Fellows_Road[m]>"
  TRAFFIC_SCHEDULER/10 -> Bus Creator3/6, ASMSignalBusCollect/4(v_Fellows_In[km|h])  "v_Fellows_Ref_Scheduler[km|h]"
  Customize_UserSignals/1(ASMSignalBus) -> [ASMBUS_Traffic_UserSignals_Customized]
  Objects_Signals/1 -> Bus Selector7/1
  Bus Creator3/1 -> Fellows_Signals/1  "FellowMovement"
  Bus Creator1/1 -> Traffic_Signals_toRoad/1
  Bus Selector7/2 -> FELLOW_POSITIONS/2  "<Wheel_Radius_Fellows[m]>"
  Bus Selector7/1 -> FELLOW_POSITIONS/1  "<Length_Fellows[m]>"
  Bus Selector5/6 -> Signal Specification5/1  "<Angle_Roll_Fellows_Road[deg]>"
  Bus Selector5/5 -> Signal Specification4/1  "<Angle_Pitch_Fellows_Road[deg]>"
  Bus Selector5/4 -> Signal Specification3/1  "<Angle_Yaw_Fellows_Road[deg]>"
  Bus Selector5/3 -> Signal Specification2/1  "<Pos_z_Fellows_Road[m]>"
  Bus Selector5/2 -> Signal Specification1/1  "<Pos_y_Fellows_Road[m]>"
  Bus Selector5/1 -> Signal Specification/1  "<Pos_x_Fellows_Road[m]>"
  TRAFFIC_SCHEDULER/6 -> Bus Creator1/5  "v_Lat_Fellows_Ref_Scheduler[m|s]"
  TRAFFIC_SCHEDULER/5 -> Bus Creator1/4  "ForceToRoad_Fellows_Ref_Scheduler[0|1]"
  TRAFFIC_SCHEDULER/4 -> Bus Creator1/3  "LaneIdx_Fellows_Ref_Scheduler[]"
  TRAFFIC_SCHEDULER/13 -> LabelUserSignals/1(UserSignals_In)
  Bus Selector1/2 -> AvoidAlgLoop_v_Fellows2/1  "<LaneIdx_Total_Fellows_Road[]>"
  Bus Selector1/1 -> AvoidAlgLoop_v_Fellows1/1  "<d_Total_Fellows_Road[m]>"
  Bus Selector3/3 -> AvoidAlgLoop_d_Road1/1  "<LaneIdx_Total_Veh_Road[]>"
  [TAG_Sw_TrafficEnable] -> TRAFFIC_SCHEDULER/1
  Bus Selector4/1 -> AvoidAlgLoop_s_Vehicle/1  "<s_Vehicle[m]>"
  TRAFFIC_SCHEDULER/3 -> Bus Creator1/2  "d_Fellows_Ref_Scheduler[m]"
  TRAFFIC_SCHEDULER/2 -> Bus Creator1/1, Bus Creator3/5, ASMSignalBusCollect/3(s_Fellows_Road[m])  "s_Fellows_Ref_Scheduler[m]"
  Bus Selector3/1 -> AvoidAlgLoop_s_Road/1  "<s_Veh_Road_Trj[m]>"
  Bus Selector2/2 -> AvoidAlgLoop_s_Road2/1  "<ManeuverTime[s]>"
  Bus Selector2/1 -> Maneuver_Status_Handling/1(ManeuverState[])  "<ManeuverState[]>"
  Maneuver_Status_Handling/1(Traffic_Ctrl) -> AvoidAlgLoop_s_Road1/1
  Bus Selector3/2 -> AvoidAlgLoop_d_Road/1  "<d_Total_Veh_Road[m]>"
  Maneuver_Signals/1 -> Bus Selector2/1, Bus Selector13/1, Bus Selector6/1
  Road_Signals/1 -> Bus Selector10/1, Bus Selector1/1, Bus Selector8/1, Bus Selector3/1, Bus Selector5/1
  TRAFFIC_SCHEDULER/7 -> Bus Creator1/6  "Direction_Fellows_Ref_Scheduler[-1|1]"
  TRAFFIC_SCHEDULER/12 -> Bus Creator3/7, FELLOW_VELOCITIES/4, FELLOW_POSITIONS/10, Bus Creator1/9  "Flag_FellowUsed[0|1]"
  TRAFFIC_SCHEDULER/8 -> Bus Creator1/7  "Route_Id_Fellows_Ref_Scheduler[]"
  TRAFFIC_SCHEDULER/9 -> Bus Creator1/8  "Dist_Def_Trf[]"
  Bus Selector1/4 -> AvoidAlgLoop_v_Fellows3/1  "<Distance_xy[m]>"
  Bus Selector1/3 -> Sw_SpeedLimit_Enable/1(SpeedLimit_In)  "<Speed_Limit_Fellows[]>"
  Sw_SpeedLimit_Enable/1(SpeedLimit_Out) -> AvoidAlgLoop_v_Fellows4/1
  Signal Specification/1 -> FELLOW_POSITIONS/3
  Signal Specification1/1 -> FELLOW_POSITIONS/4
  Signal Specification2/1 -> FELLOW_POSITIONS/5
  Signal Specification3/1 -> FELLOW_POSITIONS/6
  Signal Specification4/1 -> FELLOW_POSITIONS/7
  Signal Specification5/1 -> FELLOW_POSITIONS/8
  TRAFFIC_SCHEDULER/14 -> LabelUserSignals_Fellows/1(UserSignals_In)
  TRAFFIC_SCHEDULER/15 -> Bus Creator3/13
  TRAFFIC_SCHEDULER/11 -> FELLOW_POSITIONS/9  "Angle_Yaw_Fellows_Ref_Scheduler[deg]"

== system ASM_Traffic_V2X_Complete_Model_2/MDL/Environment/Traffic/ObjectParameters ==
  Maneuver_Signals : Inport
  ASMSignalCollector : Subsystem
  Bus Creator : BusCreator  Inputs=4
  Bus Creator1 : BusCreator  Inputs=7
  Bus Selector : BusSelector  OutputSignals=MdlControl.RoadControl[]
  DISCRETE_OBJECTS : ASM_Traffic_lib/Objects/DISCRETE_OBJECTS  Tag=ASM_SUBCOMPONENT  DiscreteObjects_1=MDL.Traffic.DiscreteObjects.DiscreteObjects_1  DiscreteObjects_2=MDL.Traffic.DiscreteObjects.DiscreteObjects_2  DiscreteObjects_3=MDL.Traffic.DiscreteObjects.DiscreteObjects_3  DiscreteObjects_4=MDL.Traffic.DiscreteObjects.DiscreteObjects_4  DiscreteObjects_5=MDL.Traffic.DiscreteObjects.DiscreteObjects_5  DiscreteObjects_6=MDL.Traffic.DiscreteObjects.DiscreteObjects_6  Const_Length_Bounding_Rectangle_Quadrant=MDL.Traffic.DiscreteObjects.Const_Length_Bounding_Rectangle_Quadrant  ASMProperties=struct('Name','DISCRETE_OBJECTS','Version','3.0','Library','ASM_Traffic_lib')  ASMInstanceName=discrete_objects  ASMInstanceID=1
  FELLOW_PARAMETERS : ASM_Traffic_lib/Objects/FELLOW_PARAMETERS  Tag=ASM_SUBCOMPONENT  TrafficObject_Type_Fellows=MDL.Traffic.Sensors.Fellows.TrafficObject_Type_Fellows  ASMProperties=struct('Name','FELLOW_PARAMETERS','Version','10.0','Library','ASM_Traffic_lib')  ASMInstanceName=fellow_parameters  ASMInstanceID=1
  Object_Reload_Trigger : Subsystem
  TRAFFIC_OBJECTS : ASM_Traffic_lib/Objects/TRAFFIC_OBJECTS  Tag=ASM_SUBCOMPONENT  ObjRoad_1=MDL.Traffic.Objects.RoadObjects_1  ObjRoad_2=MDL.Traffic.Objects.RoadObjects_2  ObjRoad_3=MDL.Traffic.Objects.RoadObjects_3  ObjRoad_4=MDL.Traffic.Objects.RoadObjects_4  ObjRoad_5=MDL.Traffic.Objects.RoadObjects_5  ObjRoad_6=MDL.Traffic.Objects.RoadObjects_6  ObjTraffic=MDL.Traffic.Objects.TrafficObjects  ASMProperties=struct('Name','TRAFFIC_OBJECTS','Version','4.0','Library','ASM_Traffic_lib')  ASMInstanceName=traffic_objects  ASMInstanceID=1
  Objects_Signals : Outport
  tag scope: ASMBUS_Environment_Traffic_DiscreteObjects=global, ASMBUS_Environment_Traffic_FellowParameters=global, ASMBUS_Environment_Traffic_TrafficObjects=global
  wires:
  Object_Reload_Trigger/1(Ctrl) -> TRAFFIC_OBJECTS/2, DISCRETE_OBJECTS/2
  DISCRETE_OBJECTS/2 -> Bus Creator/4  "DiscreteObject_Data[]"
  DISCRETE_OBJECTS/1 -> [ASMBUS_Environment_Traffic_DiscreteObjects]
  FELLOW_PARAMETERS/9 -> Bus Creator/2  "TrafficObject_Type_Fellows[]"
  FELLOW_PARAMETERS/2 -> Bus Creator1/1
  TRAFFIC_OBJECTS/1 -> [ASMBUS_Environment_Traffic_TrafficObjects]
  Bus Selector/1 -> Object_Reload_Trigger/1(RoadCtrl[])  "<RoadControl[]>"
  Maneuver_Signals/1 -> Bus Selector/1
  [TAG_Sw_RoadSelect] -> DISCRETE_OBJECTS/1, TRAFFIC_OBJECTS/1
  TRAFFIC_OBJECTS/2 -> Bus Creator/3, FELLOW_PARAMETERS/1  "TrafficObject_Type_Data[]"
  Bus Creator/1 -> Objects_Signals/1  "Objects_Signals"
  FELLOW_PARAMETERS/5 -> Bus Creator1/4
  FELLOW_PARAMETERS/4 -> Bus Creator1/3
  FELLOW_PARAMETERS/1 -> [ASMBUS_Environment_Traffic_FellowParameters]
  Bus Creator1/1 -> Bus Creator/1  "FellowsGeometry"
  FELLOW_PARAMETERS/8 -> Bus Creator1/7
  FELLOW_PARAMETERS/7 -> Bus Creator1/6
  FELLOW_PARAMETERS/6 -> Bus Creator1/5
  FELLOW_PARAMETERS/3 -> Bus Creator1/2

== system ASM_Traffic_V2X_Complete_Model_2/MDL/Environment/Traffic/Sensors ==
  Fellows_Signals : Inport
  VehicleDynamics_Signals : Inport  Port=2
  Objects_Signals : Inport  Port=3
  Road_Signals : Inport  Port=4
  Maneuver_Signals : Inport  Port=5
  ASMSignalCollector : Subsystem
  Bus Creator : BusCreator  Inputs=6
  Collision_Sensor : Subsystem
  Custom_Sensor : Subsystem
  Line_Sensor : Subsystem
  Object_Sensor_2D : Subsystem
  Object_Sensor_3D : Subsystem
  Sensors_Common_Signals : Subsystem
  Traffic_Sign_Sensor : Subsystem
  Sensor_Signals : Outport
  tag scope: ASMBUS_Environment_Traffic_Sensors_Common=global
  wires:
  Collision_Sensor/1(Sensor_Signals) -> Bus Creator/6  "Collision_Sensor"
  Fellows_Signals/1 -> Custom_Sensor/1(Fellows_Signals), Collision_Sensor/2(Fellows_Signals), Object_Sensor_2D/2(Fellows_Signals), Object_Sensor_3D/2(Fellows_Signals)
  Line_Sensor/1(Sensor_Signals) -> Bus Creator/5  "Line_Sensor"
  Maneuver_Signals/1 -> Sensors_Common_Signals/1(Maneuver_Signals[]), Line_Sensor/4(Maneuver_Signals), Collision_Sensor/6(Maneuver_Signals)
  Sensors_Common_Signals/2(Enable_Sensor_Scheduling[0Off|1On]) -> Object_Sensor_3D/1(Enable[0Off|1On]), Object_Sensor_2D/1(Enable[0Off|1On]), Line_Sensor/1(Enable[0Off|1On]), Collision_Sensor/1(Enable[0Off|1On])
  Sensors_Common_Signals/1(ASMSignalBus) -> [ASMBUS_Environment_Traffic_Sensors_Common]
  Bus Creator/1 -> Sensor_Signals/1  "Sensors"
  Custom_Sensor/1(Sensor_Signals) -> Bus Creator/3  "Custom_Sensor"
  Traffic_Sign_Sensor/1(Sensor_Signals) -> Bus Creator/4  "Traffic_Sign_Sensor"
  Object_Sensor_2D/1(Sensor_Signals) -> Bus Creator/2  "Object_Sensor_2D"
  Road_Signals/1 -> Object_Sensor_3D/5(Road_Signals), Custom_Sensor/4(Road_Signals), Traffic_Sign_Sensor/3(Road_Signals), Line_Sensor/3(Road_Signals), Collision_Sensor/5(Road_Signals), Object_Sensor_2D/5(Road_Signals)
  Objects_Signals/1 -> Custom_Sensor/3(Objects_Signals), Collision_Sensor/4(Objects_Signals), Traffic_Sign_Sensor/2(Objects_Signals), Object_Sensor_2D/4(Objects_Signals), Object_Sensor_3D/4(Objects_Signals)
  VehicleDynamics_Signals/1 -> Custom_Sensor/2(VehicleDynamics_Signals), Traffic_Sign_Sensor/1(VehicleDynamics_Signals), Collision_Sensor/3(VehicleDynamics_Signals), Line_Sensor/2(VehicleDynamics_Signals), Object_Sensor_2D/3(VehicleDynamics_Signals), Object_Sensor_3D/3(VehicleDynamics_Signals)
  Object_Sensor_3D/1(Sensor_Signals) -> Bus Creator/1  "Object_Sensor_3D"

== system ASM_Traffic_V2X_Complete_Model_2/MDL/SoftECU/ASMSignalCollector/ChangeLabel ==
  In : Inport
  Out : Outport
  wires:
  In/1 -> Out/1  "SoftECU_StartButton"

== system ASM_Traffic_V2X_Complete_Model_2/MDL/SoftECU/Map_Inputs/Maneuver ==
  note: Initial value is set
      | to ESP (2)
  note: Initial value is set
      | to ASR On (1)
  ECU_Commands[] : Inport
  Reset[0|1] : Inport  Port=2
  Add : Sum  Inputs=+++
  Data Type Conversion : DataTypeConversion
  Data Type Conversion1 : DataTypeConversion
  Fcn10 : Fcn  Expr=u(1)==2011
  Fcn2 : Fcn  Expr=u(1)==2010
  Fcn3 : Fcn  Expr=u(1)==2021
  Fcn4 : Fcn  Expr=u(1)==2020
  Fcn9 : Fcn  Expr=u(1)==2012
  Gain : Gain  Gain=0
  Gain1 : Gain
  Gain2 : Gain  Gain=2
  Logical Operator1 : Logic  Operator=OR  AllPortsSameDT=off  OutDataTypeStr=boolean
  Logical Operator2 : Logic  AllPortsSameDT=off  OutDataTypeStr=boolean
  Logical Operator3 : Logic  Operator=NOT  Inputs=1  AllPortsSameDT=off  OutDataTypeStr=boolean
  Logical Operator : Logic  Operator=OR  Inputs=4  AllPortsSameDT=off  OutDataTypeStr=boolean
  Memory : Memory  InitialCondition=2
  S_R_FlipFlop : Subsystem  mask(S_R_FlipFlop){initial_condition=1}
      mask prompts: initial_condition "Initial condition (state of Q):"
      mask help: S-R Flip-Flop Block
  Sw_ESP_Default : Constant  Value=2
  Switch : Switch  Threshold=0.5
  Switch1 : Switch  Threshold=0.5
  Terminator : Terminator
  pos_edge_detection : Subsystem
  pos_edge_detection1 : Subsystem
  pos_edge_detection2 : Subsystem
  pos_edge_detection3 : Subsystem
  Sw_ESP[0Off|1ABS|2ESP] : Outport
  Sw_ASR0Off|1On] : Outport  Port=2
  wires:
  Fcn3/1 -> Logical Operator2/2
  Logical Operator3/1 -> Logical Operator2/1
  Logical Operator2/1 -> Data Type Conversion1/1
  Data Type Conversion1/1 -> S_R_FlipFlop/2(R)
  Data Type Conversion/1 -> S_R_FlipFlop/1(S)
  ECU_Commands[]/1 -> Fcn3/1, Fcn4/1, Fcn9/1, Fcn10/1, Fcn2/1
  Fcn9/1 -> pos_edge_detection/1(In1), Gain2/1
  Fcn10/1 -> pos_edge_detection1/1(In1), Gain1/1
  Fcn2/1 -> pos_edge_detection2/1(In1), Gain/1
  pos_edge_detection/1(Out1) -> Logical Operator/1
  pos_edge_detection1/1(Out1) -> Logical Operator/2
  pos_edge_detection2/1(Out1) -> Logical Operator/3
  Gain2/1 -> Add/3
  Gain1/1 -> Add/2
  Gain/1 -> Add/1
  Logical Operator/1 -> Switch/2
  Switch/1 -> Sw_ESP[0Off|1ABS|2ESP]/1, Memory/1
  Memory/1 -> Switch/3
  pos_edge_detection3/1(Out1) -> Switch1/2, Logical Operator/4
  Add/1 -> Switch1/3
  Reset[0|1]/1 -> Logical Operator1/1, Logical Operator3/1, pos_edge_detection3/1(In1)
  Switch1/1 -> Switch/1
  Sw_ESP_Default/1 -> Switch1/1
  S_R_FlipFlop/1(Q) -> Sw_ASR0Off|1On]/1
  Fcn4/1 -> Logical Operator1/2
  Logical Operator1/1 -> Data Type Conversion/1
  S_R_FlipFlop/2(!Q) -> Terminator/1

== system ASM_Traffic_V2X_Complete_Model_2/MDL/SoftECU/Soft_ECU_ACC/ASMSignalCollector ==
  BusCreator1 : BusCreator  Inputs=4
  ASMSignalBus : Outport
  wires:
  [ASMBUS_SoftECU_ACC_Target_Selection] -> BusCreator1/4
  [ASMBUS_SoftECU_ACC_User_Interface] -> BusCreator1/3
  BusCreator1/1 -> ASMSignalBus/1  "SoftECU_ACC"
  [ASMBUS_SoftECU_ACC_Interface] -> BusCreator1/2
  [ASMBUS_SoftECU_ACC_Controller] -> BusCreator1/1

== system ASM_Traffic_V2X_Complete_Model_2/MDL/SoftECU/Soft_ECU_ACC/Input_Selection ==
  PosVec_MainPnt_In : Inport
  Reshape1 : Reshape  OutputDimensions=[]
  Selector1 : Selector  NumberOfDimensions=2  InputPortWidth=15  IndexOptions=Index vector (dialog),Index vector (dialog)  Indices=[1:15],1  OutputSizes=1,1
  PosVec_MainPnt_Out : Outport
  wires:
  Reshape1/1 -> PosVec_MainPnt_Out/1
  Selector1/1 -> Reshape1/1
  PosVec_MainPnt_In/1 -> Selector1/1

== system ASM_Traffic_V2X_Complete_Model_2/MDL/SoftECU/Soft_ECU_ACC/Map_Inputs ==
  Reset[0|1] : Inport
  Switches_ACC_User : Inport  Port=2
  ECU_Commands[] : Inport  Port=3
  Bus Selector2 : BusSelector  OutputSignals=Sw_ACC_Control_Mode[1ManSched|2Manual],Sw_ACC_On[Off|1On],Sw_ACC_Off[0Off|1On],Sw_ACC_Cancel[0Off|1On],Sw_ACC_Resume[0Off|1On],Sw_ACC_Speed_Set[0Off|1On],Sw_ACC_Speed_Increase[0Off|1On],Sw_ACC_Speed_Decrease[0Off|1On],Sw_ACC_BrakeMode[1Comfort|2AEBOnly|3AEBOff]
  Maneuver : Subsystem
  Multiport Switch{1..8} (8 alike) : MultiPortSwitch  Inputs=2  SaturateOnIntegerOverflow=on
  Sw_ACC_On[0Off|1On] : Outport
  Sw_ACC_Off[0Off|1On] : Outport  Port=2
  Sw_ACC_Cancel[0Off|1On] : Outport  Port=3
  Sw_ACC_Resume[0Off|1On] : Outport  Port=4
  Sw_ACC_Speed_Set[0Off|1On] : Outport  Port=5
  Sw_ACC_Speed_Increase[0Off|1On] : Outport  Port=6
  Sw_ACC_Speed_Decrease[0Off|1On] : Outport  Port=7
  Sw_ACC_BrakeMode[1Comfort|2AEBOnly|3AEBOff] : Outport  Port=8
  wires:
  Multiport Switch7/1 -> Sw_ACC_On[0Off|1On]/1
  Multiport Switch6/1 -> Sw_ACC_Off[0Off|1On]/1
  Multiport Switch4/1 -> Sw_ACC_Cancel[0Off|1On]/1
  Multiport Switch3/1 -> Sw_ACC_Resume[0Off|1On]/1
  Multiport Switch5/1 -> Sw_ACC_Speed_Set[0Off|1On]/1
  Multiport Switch2/1 -> Sw_ACC_Speed_Increase[0Off|1On]/1
  Multiport Switch1/1 -> Sw_ACC_Speed_Decrease[0Off|1On]/1
  Switches_ACC_User/1 -> Bus Selector2/1
  ECU_Commands[]/1 -> Maneuver/1(ECU_Commands[])
  Bus Selector2/1 -> Multiport Switch7/1, Multiport Switch6/1, Multiport Switch4/1, Multiport Switch3/1, Multiport Switch5/1, Multiport Switch2/1, Multiport Switch8/1, Multiport Switch1/1  "<Sw_ACC_Control_Mode[1ManSched|2Manual]>"
  Bus Selector2/2 -> Multiport Switch7/3  "<Sw_ACC_On[Off|1On]>"
  Bus Selector2/3 -> Multiport Switch6/3  "<Sw_ACC_Off[0Off|1On]>"
  Bus Selector2/4 -> Multiport Switch4/3  "<Sw_ACC_Cancel[0Off|1On]>"
  Bus Selector2/5 -> Multiport Switch3/3  "<Sw_ACC_Resume[0Off|1On]>"
  Bus Selector2/6 -> Multiport Switch5/3  "<Sw_ACC_Speed_Set[0Off|1On]>"
  Bus Selector2/7 -> Multiport Switch2/3  "<Sw_ACC_Speed_Increase[0Off|1On]>"
  Bus Selector2/8 -> Multiport Switch1/3  "<Sw_ACC_Speed_Decrease[0Off|1On]>"
  Maneuver/1(Sw_ACC_On[0Off|1On]) -> Multiport Switch7/2
  Maneuver/2(Sw_ACC_Off[0Off|1On]) -> Multiport Switch6/2
  Maneuver/3(Sw_ACC_Cancel[0Off|1On]) -> Multiport Switch4/2
  Maneuver/4(Sw_ACC_Resume[0Off|1On]) -> Multiport Switch3/2
  Maneuver/5(Sw_ACC_Speed_Set[0Off|1On]) -> Multiport Switch5/2
  Maneuver/6(Sw_ACC_Speed_Increase[0Off|1On]) -> Multiport Switch2/2
  Maneuver/7(Sw_ACC_Speed_Decrease[0Off|1On]) -> Multiport Switch1/2
  Reset[0|1]/1 -> Maneuver/2(Reset[0|1])
  Multiport Switch8/1 -> Sw_ACC_BrakeMode[1Comfort|2AEBOnly|3AEBOff]/1
  Maneuver/8(Sw_ACC_BrakeMode[1Comfort|2AEBOnly|3AEBOff]) -> Multiport Switch8/2
  Bus Selector2/9 -> Multiport Switch8/3  "<Sw_ACC_BrakeMode[1Comfort|2AEBOnly|3AEBOff]>"

== system ASM_Traffic_V2X_Complete_Model_2/MDL/SoftECU/Soft_ECU_ACC/Tire ==
  Tire : Inport
  Bus Selector1 : BusSelector  OutputSignals=Tire_FL.ActiveTire.r_Dyn_FL_Tire[m],Tire_FR.ActiveTire.r_Dyn_FR_Tire[m],Tire_RL.ActiveTire.r_Dyn_RL_Tire[m],Tire_RR.ActiveTire.r_Dyn_RR_Tire[m],Tire_FL.ActiveTire.Coef_RollingRes_FL[],Tire_FR.ActiveTire.Coef_RollingRes_FR[],Tire_RL.ActiveTire.Coef_RollingRes_RL[],Tire_RR.ActiveTire.Coef_RollingRes_RR[]
  Coef_RolRes_Mean : Fcn  Expr=(u(1)+u(2)+u(3)+u(4))/4
  Mux : Mux
  Mux1 : Mux
  r_Dyn_Tire_Mean : Fcn  Expr=(u(1)+u(2)+u(3)+u(4))/4
  r_Dyn_Tire_Mean[m] : Outport
  Coef_RollingRes_Mean[] : Outport  Port=2
  wires:
  Coef_RolRes_Mean/1 -> Coef_RollingRes_Mean[]/1
  r_Dyn_Tire_Mean/1 -> r_Dyn_Tire_Mean[m]/1
  Bus Selector1/8 -> Mux1/4  "<Coef_RollingRes_RR[]>"
  Bus Selector1/7 -> Mux1/3  "<Coef_RollingRes_RL[]>"
  Bus Selector1/6 -> Mux1/2  "<Coef_RollingRes_FR[]>"
  Bus Selector1/5 -> Mux1/1  "<Coef_RollingRes_FL[]>"
  Bus Selector1/4 -> Mux/4  "<r_Dyn_RR_Tire[m]>"
  Bus Selector1/3 -> Mux/3  "<r_Dyn_RL_Tire[m]>"
  Bus Selector1/2 -> Mux/2  "<r_Dyn_FR_Tire[m]>"
  Bus Selector1/1 -> Mux/1  "<r_Dyn_FL_Tire[m]>"
  Mux/1 -> r_Dyn_Tire_Mean/1
  Mux1/1 -> Coef_RolRes_Mean/1
  Tire/1 -> Bus Selector1/1

== system ASM_Traffic_V2X_Complete_Model_2/MDL/SoftECU/Soft_ECU_ACC/TrackWidthVehicle ==
  Pos_FL_Wheel[x;y;z][m] : Inport
  Pos_FR_Wheel[x;y;z][m] : Inport  Port=2
  Abs : Abs
  Abs1 : Abs
  Add : Sum
  Selector : Selector  InputPortWidth=3  IndexOptions=Index vector (dialog)  Indices=[2]  OutputSizes=1
  TrackWidth_Vehicle[m] : Outport
  wires:
  Pos_FR_Wheel[x;y;z][m]/1 -> Abs1/1
  Pos_FL_Wheel[x;y;z][m]/1 -> Abs/1
  Selector/1 -> TrackWidth_Vehicle[m]/1
  Add/1 -> Selector/1
  Abs1/1 -> Add/2
  Abs/1 -> Add/1

== system ASM_Traffic_V2X_Complete_Model_2/MDL/SoftECU/Soft_ECU_Brake/ASMSignalCollector ==
  Bus Creator : BusCreator  Inputs=1
  ASMSignalBus : Outport
  wires:
  Bus Creator/1 -> ASMSignalBus/1  "SoftECU_Brake"
  [ASMBUS_SoftECU_BrakeDesired] -> Bus Creator/1

== system ASM_Traffic_V2X_Complete_Model_2/MDL/SoftECU/Soft_ECU_Engine_Basic/ASMSignalCollector ==
  Bus Creator : BusCreator  Inputs=4
  ASMSignalBus : Outport
  wires:
  [ASMBUS_SoftECU_Engine_EngineOperation] -> Bus Creator/4
  Bus Creator/1 -> ASMSignalBus/1  "SoftECU_Engine"
  [ASMBUS_SoftECU_Engine_TorqueIntervention_fast] -> Bus Creator/1
  [ASMBUS_SoftECU_Engine_TorqueIntervention_slow] -> Bus Creator/2
  [ASMBUS_SoftECU_Engine_IdleSpeedControl] -> Bus Creator/3

== system ASM_Traffic_V2X_Complete_Model_2/MDL/SoftECU/Soft_ECU_Engine_Basic/DisableReset ==
  note: No start request will be sent, if the engine has not been reset
  Reset_VehicleStates[0|1] : Inport
  MultiPortSwitch : MultiPortSwitch  DataPortOrder=Zero-based contiguous  Inputs=2  zeroidx=on  SaturateOnIntegerOverflow=on  InputSameDT=on
  NO_Reset : Constant  Value=0
  Reset[0|1] : Outport
  wires:
  Reset_VehicleStates[0|1]/1 -> MultiPortSwitch/3
  NO_Reset/1 -> MultiPortSwitch/2
  [TAG_Drivetrain_Sw_CrankShaft_Reset] -> MultiPortSwitch/1
  MultiPortSwitch/1 -> Reset[0|1]/1
